simulink model "mpcLearning"  (R2021a)
settings: Solver=VariableStepAuto  StartTime=0.0  StopTime=20  RelTol=1e-3
values from neighbouring files (symbols this model uses):
  b = 1.2    [mpcEffort.m]
  k = 1    [mpcEffort.m]
  m = 1    [mpcEffort.m]
  sys = linearize(plant_mdl)    [mpcEffort.m]    (also in mpcwork.m = sys(:,2:3))
  Ts = 0.1    [mpcEffort.m]    (also in mpcwork.m = 0.5)
libraries: mpclib x1, simulink x1
settings Model: Creator=golam  LastModifiedBy=jamagola
settings SolverCC: AlgebraicLoopSolver=TrustRegion
settings DebuggingCC: SFMachineParentedDataDiag=warning

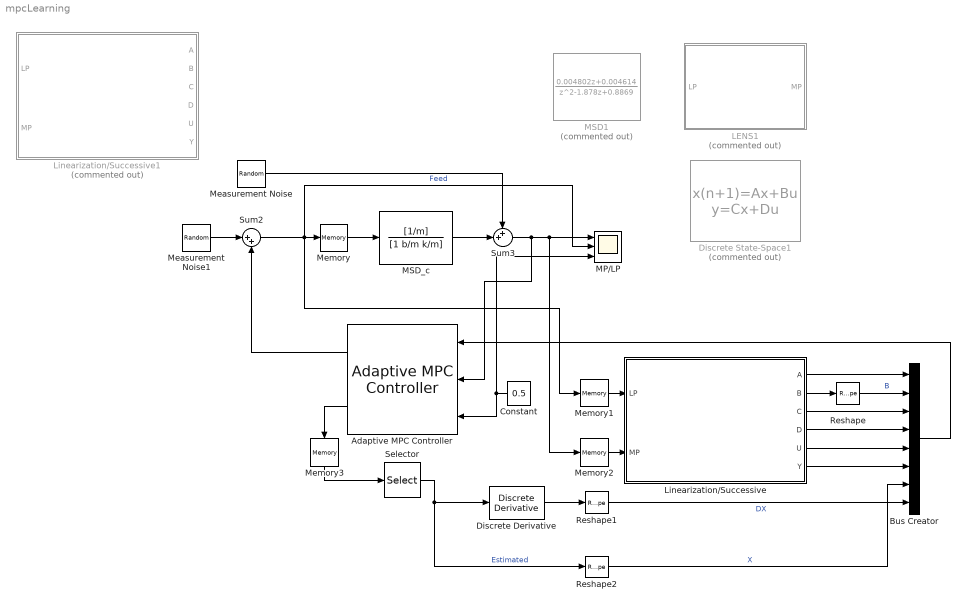
== system mpcLearning ==
  Adaptive MPC Controller : mpclib/Adaptive MPC Controller  SCDEnableBlockLinearizationSpecification=on  mpcobj=mpcobj  enable_value=0  updateMPCinCallerWorkspace=on  md_inport=off  mv_inport=off  uref_inport=off  return_cost=off  return_mvseq=off  return_qpstatus=off  return_xseq=off  return_state=on  return_ovseq=off  state_inport=off  isltv_plant=off  umin_inport=off  umax_inport=off  ymin_inport=off  ymax_inport=off  cc_inport=off  ywt_inport=off  uwt_inport=off  duwt_inport=off  rhoeps_inport=off  pm_inport=off  MaximumP=10  HorizonChoice=FixedHorizon  BlockDataType=double  SampleTimeInherited=off  switch_inport=off
      settings: SourceProductName=Model Predictive Control Toolbox
  Bus Creator : BusCreator  Inputs=8
  Constant : Constant  Value=0.5  SampleTime=Ts
  Discrete Derivative : simulink/Discrete/Discrete Derivative  gainval=1.0  ICPrevScaledInput=0.0  InputProcessing=Columns as channels (frame based)  OutMin=[]  OutMax=[]  OutDataType=fixdt(1, 16)  OutScaling=2^-10  DoSatur=off
  Discrete State-Space1 : DiscreteStateSpace  Commented=on  A=sys.A  B=sys.B  C=sys.C  D=sys.D  SampleTime=Ts
  LENS1 : Subsystem  Commented=on
  Linearization/Successive : MATLAB Function  TreatAsAtomicUnit=on
  Linearization/Successive1 : MATLAB Function  Commented=on  TreatAsAtomicUnit=on
  MP/LP : Scope  NumInputPorts=3
  MSD1 : DiscreteTransferFcn  Commented=on  Numerator=[0.004802 0.004614]  Denominator="[1.0000   -1.878    0.8869]"  SampleTime=0.1
  MSD_c : TransferFcn  Numerator=[1/m]  Denominator=[1 b/m k/m]
  Measurement Noise : RandomNumber  Mean=[0]  Variance=0.001*[1]  Seed=98325  SampleTime=Ts
  Measurement Noise1 : RandomNumber  Mean=[0]  Variance=0*[1]  Seed=98325  SampleTime=Ts
  Memory{,1..3} (4 alike) : Memory  InheritSampleTime=on  LinearizeAsDelay=on
  Reshape : Reshape  OutputDimensionality=Customize  OutputDimensions=[2,1]
  Reshape1 : Reshape  OutputDimensionality=Customize  OutputDimensions=[2,1]
  Reshape2 : Reshape  OutputDimensionality=Customize  OutputDimensions=[2,1]
  Selector : Selector  InputPortWidth=3  IndexOptions=Index vector (dialog)  Indices=[1:2]  OutputSizes=1
  Sum2 : Sum  Inputs=|++  SampleTime=Ts/5
  Sum3 : Sum  Inputs=++|  SampleTime=Ts/5
  wires:
  MSD_c/1 -> Sum3/2
  Constant/1 -> Adaptive MPC Controller/3, MP/LP/3
  Measurement Noise/1 -> Sum3/1
  Adaptive MPC Controller/1 -> Sum2/2
  Sum2/1 -> Memory/1, MP/LP/2, Memory1/1  "Feed"
  Measurement Noise1/1 -> Sum2/1
  Linearization/Successive/1(A) -> Bus Creator/1
  Linearization/Successive/2(B) -> Reshape/1
  Linearization/Successive/3(C) -> Bus Creator/3
  Linearization/Successive/4(D) -> Bus Creator/4
  Linearization/Successive/5(U) -> Bus Creator/5
  Linearization/Successive/6(Y) -> Bus Creator/6
  Sum3/1 -> Memory2/1, MP/LP/1, Adaptive MPC Controller/2
  Bus Creator/1 -> Adaptive MPC Controller/1
  Reshape2/1 -> Bus Creator/7  "X"
  Reshape1/1 -> Bus Creator/8  "DX"
  Reshape/1 -> Bus Creator/2  "B"
  Memory/1 -> MSD_c/1
  Memory1/1 -> Linearization/Successive/1(LP)
  Memory2/1 -> Linearization/Successive/2(MP)
  Adaptive MPC Controller/2 -> Memory3/1
  Discrete Derivative/1 -> Reshape1/1
  Selector/1 -> Reshape2/1, Discrete Derivative/1  "Estimated"
  Memory3/1 -> Selector/1

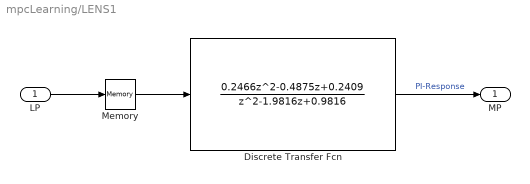
== system mpcLearning/LENS1 ==
  LP : Inport
  Discrete Transfer Fcn : DiscreteTransferFcn  Numerator="[0.2466   -0.4875    0.2409]"  Denominator="[1.0000   -1.9816    0.9816]"  SampleTime=0.1
  Memory : Memory  InheritSampleTime=on  LinearizeAsDelay=on
  MP : Outport
  wires:
  Discrete Transfer Fcn/1 -> MP/1  "PI-Response"
  LP/1 -> Memory/1
  Memory/1 -> Discrete Transfer Fcn/1

== matlab function mpcLearning/Linearization//Successive ==
  data: LP input; A output; MP input; B output; C output; D output; U output; Y output
function [A, B, C, D, U, Y] = fcn(LP,MP)
% test
% num=[0.2466 0.05715 0.001018];
% den=[1 0.1855 0.003452];
% Ts=0.1;
% H=tf(num,den);
% H_d=c2d(H,Ts);
% n=cell2mat(H_d.num);
% d=cell2mat(H_d.den);

%plant_mdl = 'amplant';
%sys = linearize(plant_mdl);
%sys=minreal(sys);


A=[0.995 0.0998; -0.0998 0.9950];
B=[0.004996 0.09983]';
C=[0 1];
% A=[0.1372, -0.8444; -0.1372, 0.8444];
% B=[-0.7071, -0.7071]';
% C=[-0.1732, -0.1755];
% A=[0 0 0; 1 1.982 -0.9816; 0 1 0];
% B=[1;0;0];
% C=[0.2466 0.001163 -0.001163];
D=[0];
U=[LP];
Y=[MP];
end

== matlab function mpcLearning/Linearization//Successive1 ==
  data: LP input; A output; MP input; B output; C output; D output; U output; Y output
function [A, B, C, D, U, Y] = fcn(LP,MP)

% num=[0.2466 0.05715 0.001018];
% den=[1 0.1855 0.003452];
% Ts=0.1;
% H=tf(num,den);
% H_d=c2d(H,Ts);
% n=cell2mat(H_d.num);
% d=cell2mat(H_d.den);

%plant_mdl = 'amplant';
%sys = linearize(plant_mdl);
%sys=minreal(sys);

A=[0.1372, -0.8444; -0.1372, 0.8444];
B=[-0.7071, -0.7071]';
C=[-0.1732, -0.1755];
% A=[0 0 0; 1 1.982 -0.9816; 0 1 0];
% B=[1;0;0];
% C=[0.2466 0.001163 -0.001163];
D=[0];
U=[LP];
Y=[MP];
end
